simulink model "RoboBoat_NEDcallv8"  (R2014a)
settings: Solver=FixedStepDiscrete  StartTime=0.0  StopTime=inf  FixedStep=.1  RelTol=1e-3
undefined symbols (not defined in the file): Com1, Com2, Com3, Com4, DiscIntNeverNeededParam, standard
libraries: xpcseriallib x31, visiontextngfix x25, simulink x19, slrtlib x9, speedgoatlib_IO102 x3, speedgoatlib x1
(part 2 of 4)

== matlab function RoboBoat_NEDcallv8/Main FSM/Obstacle Navigation1/Obstacle Navigation/MATLAB Function ==
  data: dodgeIncomplete input; dodgeStart input; taskSelector output; dodgeEn output; GPSEn output
function [taskSelector, dodgeEn, GPSEn]  = obstNavEnabler(dodgeIncomplete, dodgeStart)

GPSEn = 0;
dodgeEn = 0;

if  dodgeStart == 1 || dodgeIncomplete == 1
    dodgeEn = 1;
    taskSelector = 1;
else
    GPSEn = 1;
    taskSelector = 2;
end

== matlab function RoboBoat_NEDcallv8/Main FSM/Obstacle Navigation1/GPS: Center/Approach/Desired Heading and Distance ==
  data: Distance output; DesiredGPS input; DesiredHeading output; GPSLat input; GPSLong input
function [Distance, DesiredHeading] = Approach(DesiredGPS, GPSLat, GPSLong)

%Written by Anderson Lebbad on July 22, 2013
%Last Edited: Edward Zhu July 5, 2014

%Edit:
% Switched from great-circle distance formula to equirectangular approx and
%used mod for desired heading
% Changed calculation to use positve lat and negative long

%Orients the boat towards a target GPS point before approaching it.
%This is done to keep the approach angle minimal, so the approach
%algorithm does not circle the target and never reach it.

%Parse input GPS and convert angles to radians
CurLat = (floor(GPSLat/100)+mod(GPSLat,100)/60)*pi/180;
CurLong = (ceil(GPSLong/100)-mod(-GPSLong,100)/60)*pi/180;
DesLat = (floor(DesiredGPS(1)/100)+mod(DesiredGPS(1),100)/60)*pi/180;
DesLong = (ceil(DesiredGPS(2)/100)-mod(-DesiredGPS(2),100)/60)*pi/180;

%Difference between lats and longs
DiffLat = DesLat - CurLat;
MidLat = cos((CurLat + DesLat)/2);
DiffLong = DesLong - CurLong;

%Radius of the earth in meters
R = 6378137;

%Calculate distance using the great-circle distance formula
%Formula documented here:
%   http://www.movable-type.co.uk/scripts/latlong.html
% a = sin(DiffLat/2)^2+sin(DiffLong/2)^2*cos(CurLat)*cos(DesLat);
% c = 2*atan2(sqrt(a), sqrt(1-a));
% Distance = R*c;

%Calculating distance using equirectangular approximation since distances
%concerned are very small
a = DiffLong*MidLat;
b = DiffLat;
Distance = R*sqrt(a^2+b^2);

%Calculate initial bearing - formula documented here: 
%   http://www.movable-type.co.uk/scripts/latlong.html
y = sin(DiffLong)*cos(DesLat);
x = cos(CurLat)*sin(DesLat)-sin(CurLat)*cos(DesLat)*cos(DiffLong);
DesiredHeading = mod(atan2(y, x)*180/pi + 360, 360);

== matlab function RoboBoat_NEDcallv8/Main FSM/Obstacle Navigation1/Obstacle Navigation/GPS: Bee Line/Approach/Desired Heading and Distance ==
  data: Distance output; DesiredGPS input; DesiredHeading output; GPSLat input; GPSLong input
function [Distance, DesiredHeading] = Approach(DesiredGPS, GPSLat, GPSLong)

%Written by Anderson Lebbad on July 22, 2013
%Last Edited: Edward Zhu July 5, 2014

%Edit:
% Switched from great-circle distance formula to equirectangular approx and
%used mod for desired heading
% Changed calculation to use positve lat and negative long

%Orients the boat towards a target GPS point before approaching it.
%This is done to keep the approach angle minimal, so the approach
%algorithm does not circle the target and never reach it.

%Parse input GPS and convert angles to radians
CurLat = (floor(GPSLat/100)+mod(GPSLat,100)/60)*pi/180;
CurLong = (ceil(GPSLong/100)-mod(-GPSLong,100)/60)*pi/180;
DesLat = (floor(DesiredGPS(1)/100)+mod(DesiredGPS(1),100)/60)*pi/180;
DesLong = (ceil(DesiredGPS(2)/100)-mod(-DesiredGPS(2),100)/60)*pi/180;

%Difference between lats and longs
DiffLat = DesLat - CurLat;
MidLat = cos((CurLat + DesLat)/2);
DiffLong = DesLong - CurLong;

%Radius of the earth in meters
R = 6378137;

%Calculate distance using the great-circle distance formula
%Formula documented here:
%   http://www.movable-type.co.uk/scripts/latlong.html
% a = sin(DiffLat/2)^2+sin(DiffLong/2)^2*cos(CurLat)*cos(DesLat);
% c = 2*atan2(sqrt(a), sqrt(1-a));
% Distance = R*c;

%Calculating distance using equirectangular approximation since distances
%concerned are very small
a = DiffLong*MidLat;
b = DiffLat;
Distance = R*sqrt(a^2+b^2);

%Calculate initial bearing - formula documented here: 
%   http://www.movable-type.co.uk/scripts/latlong.html
y = sin(DiffLong)*cos(DesLat);
x = cos(CurLat)*sin(DesLat)-sin(CurLat)*cos(DesLat)*cos(DiffLong);
DesiredHeading = mod(atan2(y, x)*180/pi + 360, 360);

== matlab function RoboBoat_NEDcallv8/Sensors/1020 Comms/Data Update2 ==
  data: Valid input; ControlMode input; V output; C output; L output; A output; Data input; D1 output; D2 output; D3 output; D4 output; D5 output; D6 output; D7 output; D8 output; D9 output; D10 output; D11 output; D12 output; D13 output; D14 output; D15 output; D16 output; D17 output; D18 output; D19 output; D20 output; D21 output; D22 output; D23 output; D24 output; Activate input
function [V,C,L,A,D1,D2,D3,D4,D5,D6,D7,D8,D9,D10,D11,D12,D13,D14,D15,D16,D17,...
    D18,D19,D20,D21,D22,D23,D24] = dataSplit(Valid,ControlMode,Data,Activate)
%Written by Anderson Lebbad on August 10, 2014
%Last Edited by: Anderson Lebbad on September 11, 2014

%This function splits the data vector into the twelve channels it is
%composed of for communication

persistent HoldData

if isempty(HoldData)
    HoldData = zeros(26,1);
    HoldData(2) = 2;
end

if Valid == 1
    HoldData(1) = Valid;
    HoldData(2) = ControlMode;
    HoldData(3) = Data(1);
    HoldData(4) = Data(2);
    HoldData(5) = Data(3);
    HoldData(6) = Data(4);
    HoldData(7) = Data(5);
    HoldData(8) = Data(6);
    HoldData(9) = Data(7);
    HoldData(10) = Data(8);
    HoldData(11) = Data(9);
    HoldData(12) = Data(10);
    HoldData(13) = Data(11);
    HoldData(14) = Data(12);
    HoldData(15) = Data(13);
    HoldData(16) = Data(14);
    HoldData(17) = Data(15);
    HoldData(18) = Data(16);
    HoldData(19) = Data(17);
    HoldData(20) = Data(18);
    HoldData(21) = Data(19);
    HoldData(22) = Data(20);
    HoldData(23) = Data(21);
    HoldData(24) = Data(22);
    HoldData(25) = Data(23);
    HoldData(26) = Data(24);
end

V = HoldData(1);
C = HoldData(2);
L = 8;
A = Activate;
D1 = HoldData(3);
D2 = HoldData(4);
D3 = HoldData(5);
D4 = HoldData(6);
D5 = HoldData(7);
D6 = HoldData(8);
D7 = HoldData(9);
D8 = HoldData(10);
D9 = HoldData(11);
D10 = HoldData(12);
D11 = HoldData(13);
D12 = HoldData(14);
D13 = HoldData(15);
D14 = HoldData(16);
D15 = HoldData(17);
D16 = HoldData(18);
D17 = HoldData(19);
D18 = HoldData(20);
D19 = HoldData(21);
D20 = HoldData(22);
D21 = HoldData(23);
D22 = HoldData(24);
D23 = HoldData(25);
D24 = HoldData(26);

end

== matlab function RoboBoat_NEDcallv8/Sensors/1020 Comms/MATLAB Function3 ==
  data: Time input; asciiHRT output; Lat input; Long input; Mode input; Task input
% This function creates the heartbeat message to be sent from Speedgoat in
% ascii code
% Written by: Edward Zhu
% Date: 9/17/14

function asciiHRT = asciiHRTEncoder(Time, Lat, Long, Mode, Task)

% Initialize output message vector as the serial output block expects 128
% character message
asciiHRT = uint8(zeros(1,128));

% Convert static strings to ascii code
asciiMsgID = uint8('$RXHRT,');
asciiComma = uint8(',');
asciiDeciPt = uint8('.');
if Lat >= 0
    asciiNS = uint8('N,');
else
    Lat = -Lat;
    asciiNS = uint8('S,');
end
if Long >= 0
    asciiEW = uint8('E,');
else
    Long = -Long;
    asciiEW = uint8('W,');
end
asciiTeamID = uint8('FAUVU,');
asciiMsgEnd = uint8('*');
asciiMsgCRLF = [13 10];

% Convert UTC Time input (hhmmss) into ascii code
asciiTime = uint8(zeros(1,7));
asciiTime(7) = asciiComma;

for timeChar = 1:6
    asciiTime(timeChar) = floor(mod(Time,10^(7-timeChar))/...
        10^(6-timeChar)) + 48;
end

% Convert latitude (dd.mmmmmm) into ascii code
asciiLat = uint8(zeros(1,10));
asciiLat(10) = asciiComma;
asciiLat(3) = asciiDeciPt;

latInt = floor(Lat);
for latIntChar = 1:2
    asciiLat(latIntChar) = floor(mod(latInt,10^(3-latIntChar))/...
        10^(2-latIntChar)) + 48;
end

latDeci = mod(Lat,latInt) * 10^6;
for latDeciChar = 1:6
    asciiLat(latDeciChar+3) = floor(mod(latDeci,10^(7-latDeciChar))/...
        10^(6-latDeciChar)) + 48;
end

% Convert longitude (ddd.mmmmmm) into ascii code
asciiLong = uint8(zeros(1,11));
asciiLong(11) = asciiComma;
asciiLong(4) = asciiDeciPt;

longInt = floor(Long);
for longIntChar = 1:3
    asciiLong(longIntChar) = floor(mod(longInt,10^(4-longIntChar))/...
        10^(3-longIntChar)) + 48;
end

longDeci = mod(Long,longInt) * 10^6;
for longDeciChar = 1:6
    asciiLong(longDeciChar+4) = floor(mod(longDeci,10^(7-longDeciChar))/...
        10^(6-longDeciChar)) + 48;
end

% Convert vehicle mode into ascii (1 = RC, 2 = Auto)
if Mode ~= 1 || Mode ~= 2
    Mode = 1;
    asciiMode = [uint8(Mode+48) asciiComma];
else
    asciiMode = [uint8(Mode+48) asciiComma];
end

% Convert vehicle task into ascii
asciiTask = [uint8(Task+48) asciiMsgEnd];

% Concat individual ascii arrays into one array
asciiPreChkSum = cat(2,asciiMsgID,asciiTime,asciiLat,asciiNS,asciiLong,asciiEW,...
    asciiTeamID,asciiMode,asciiTask);

% Calculate the checksum of the message from the '$' to the '*' and convert
% to hex
chkSum = uint8(0);

for chksumChar = 1:(length(asciiPreChkSum)-2)
    chkSum = bitxor(chkSum,asciiPreChkSum(chksumChar+1));
end

% Convert the checksum to ascii
chkSum = dec2hex(chkSum);
asciiChkSum = uint8(zeros(1,length(chkSum))+32);
for i = 1:length(chkSum)
    asciiChkSum(i) = uint8(chkSum(i));
end

% Concat the checksum and the '/r/n' to the end of the message
asciiPostChkSum = cat(2,asciiPreChkSum,asciiChkSum,asciiMsgCRLF);

% Output the final message
asciiHRT(1:length(asciiPostChkSum)) = asciiPostChkSum;

== system RoboBoat_NEDcallv8/Sensors/1020 Comms/ Raspberry Pi LCM (Navigation and Acoustics) ==
  LCM Input : Inport
  ASCII Decode 6 : xpcseriallib/ASCII Decode   format=P1:%f P2:%f P3:%f V1:%f V2:%f V3:%f E1:%f E2:%f E3:%f Pt1:%f Pt2:%f St1:%f St2:%f Start:%f Elapsed:%f RC:%d Deploy:%u, Elapsed:%g, Bearing1:%g Bearing2:%g \r\n  nvars=22  vartypes={}
  Bus Creator{,5..7} (4 alike) : BusCreator  Inputs=2
  Bus Creator{1..3,8} (4 alike) : BusCreator  Inputs=3
  Bus Creator4 : BusCreator  Inputs=9
  Data Type Conversion : DataTypeConversion  OutDataTypeStr=double
  FIFO ASCII read 1 : xpcseriallib/FIFO ASCII read   header={'P1:'}  term=[13 10]  hold=Zero output if no new data  enable=off  maxsize=2048  outputtype=8 bit uint null terminated  sampletime=-1
  Navigation LCM : Outport
  Acoustic LCM : Outport  Port=2
  wires:
  LCM Input/1 -> FIFO ASCII read 1/1
  FIFO ASCII read 1/1 -> ASCII Decode 6/1
  Bus Creator4/1 -> Navigation LCM/1  "Navigation Message"
  ASCII Decode 6/1 -> Bus Creator1/1  "X"
  ASCII Decode 6/2 -> Bus Creator1/2  "Y"
  ASCII Decode 6/3 -> Bus Creator1/3  "Psi"
  Bus Creator1/1 -> Bus Creator4/1  "Pose"
  ASCII Decode 6/4 -> Bus Creator2/1  "u"
  ASCII Decode 6/5 -> Bus Creator2/2  "v"
  Bus Creator2/1 -> Bus Creator4/2  "Velocity"
  ASCII Decode 6/7 -> Bus Creator3/1  "Roll"
  ASCII Decode 6/8 -> Bus Creator3/2  "Pitch"
  ASCII Decode 6/9 -> Bus Creator3/3  "Yaw"
  Bus Creator3/1 -> Bus Creator4/3  "Euler"
  Bus Creator5/1 -> Bus Creator4/5  "Port"
  Bus Creator6/1 -> Bus Creator4/6  "Stbd"
  ASCII Decode 6/14 -> Bus Creator6/1  "StThrust"
  ASCII Decode 6/15 -> Bus Creator6/2  "StAzimuth"
  ASCII Decode 6/12 -> Bus Creator5/1  "PtThrust"
  ASCII Decode 6/13 -> Bus Creator5/2  "PtAzimuth"
  ASCII Decode 6/16 -> Bus Creator4/7  "Start"
  ASCII Decode 6/17 -> Bus Creator4/8  "Elapsed"
  ASCII Decode 6/18 -> Data Type Conversion/1  "On/Off/RC/Auto"
  Data Type Conversion/1 -> Bus Creator4/9  "On/Off/RC/Auto"
  ASCII Decode 6/6 -> Bus Creator2/3  "r"
  ASCII Decode 6/10 -> Bus Creator7/1  "Lat"
  ASCII Decode 6/11 -> Bus Creator7/2  "Long"
  Bus Creator7/1 -> Bus Creator4/4  "GPS (LLA)"
  ASCII Decode 6/21 -> Bus Creator/1  "Horizontal Bearing"
  ASCII Decode 6/22 -> Bus Creator/2  "Vertical Bearing"
  Bus Creator/1 -> Bus Creator8/3  "Bearings"
  ASCII Decode 6/20 -> Bus Creator8/2  "Elapsed Time"
  ASCII Decode 6/19 -> Bus Creator8/1  "Deployed"
  Bus Creator8/1 -> Acoustic LCM/1  "Acoustic Message"

== system RoboBoat_NEDcallv8/Sensors/1020 Comms/ Raspberry Pi LCM (Navigation) ==
  LCM Input : Inport
  ASCII Decode 6 : xpcseriallib/ASCII Decode   format=P1:%f P2:%f P3:%f V1:%f V2:%f V3:%f E1:%f E2:%f E3:%f Lat:%f Long:%f Pt1:%f Pt2:%f St1:%f St2:%f Start:%f Elapsed:%f RC:%d Deploy:%u Elapsed:%f Bearing1:%f Bearing2:%f Range:%f X_Pos:%f Y_Pos:%f \r\n  nvars=25  vartypes={}
  Bus Creator1 : BusCreator  Inputs=3
  Bus Creator2 : BusCreator  Inputs=3
  Bus Creator3 : BusCreator  Inputs=3
  Bus Creator4 : BusCreator  Inputs=9
  Bus Creator5 : BusCreator  Inputs=2
  Bus Creator6 : BusCreator  Inputs=2
  Bus Creator7 : BusCreator  Inputs=2
  Bus Creator8 : BusCreator  Inputs=7
  Data Type Conversion : DataTypeConversion  OutDataTypeStr=double
  FIFO ASCII read 1 : xpcseriallib/FIFO ASCII read   header={'P1:'}  term=[13 10]  hold=Zero output if no new data  enable=off  maxsize=2000  outputtype=8 bit uint null terminated  sampletime=-1
  LCM Output : Outport
  Acou LCM : Outport  Port=2
  wires:
  LCM Input/1 -> FIFO ASCII read 1/1
  FIFO ASCII read 1/1 -> ASCII Decode 6/1
  Bus Creator4/1 -> LCM Output/1  "Navigation Message"
  ASCII Decode 6/1 -> Bus Creator1/1  "X"
  ASCII Decode 6/2 -> Bus Creator1/2  "Y"
  ASCII Decode 6/3 -> Bus Creator1/3  "Psi"
  Bus Creator1/1 -> Bus Creator4/1  "Pose"
  ASCII Decode 6/4 -> Bus Creator2/1  "u"
  ASCII Decode 6/5 -> Bus Creator2/2  "v"
  Bus Creator2/1 -> Bus Creator4/2  "Velocity"
  ASCII Decode 6/7 -> Bus Creator3/1  "Roll"
  ASCII Decode 6/8 -> Bus Creator3/2  "Pitch"
  ASCII Decode 6/9 -> Bus Creator3/3  "Yaw"
  Bus Creator3/1 -> Bus Creator4/3  "Euler"
  Bus Creator5/1 -> Bus Creator4/5  "Port"
  Bus Creator6/1 -> Bus Creator4/6  "Stbd"
  ASCII Decode 6/14 -> Bus Creator6/1  "StThrust"
  ASCII Decode 6/15 -> Bus Creator6/2  "StAzimuth"
  ASCII Decode 6/12 -> Bus Creator5/1  "PtThrust"
  ASCII Decode 6/13 -> Bus Creator5/2  "PtAzimuth"
  ASCII Decode 6/16 -> Bus Creator4/7  "Start"
  ASCII Decode 6/17 -> Bus Creator4/8  "Elapsed"
  ASCII Decode 6/18 -> Data Type Conversion/1  "On/Off/RC/Auto"
  Data Type Conversion/1 -> Bus Creator4/9  "On/Off/RC/Auto"
  ASCII Decode 6/6 -> Bus Creator2/3  "r"
  ASCII Decode 6/10 -> Bus Creator7/1  "Lat"
  ASCII Decode 6/11 -> Bus Creator7/2  "Long"
  Bus Creator7/1 -> Bus Creator4/4  "GPS (LLA)"
  ASCII Decode 6/19 -> Bus Creator8/1  "Deployed"
  ASCII Decode 6/20 -> Bus Creator8/2  "Elapsed Time"
  ASCII Decode 6/21 -> Bus Creator8/3  "Horizontal Bearing"
  ASCII Decode 6/22 -> Bus Creator8/4  "Vertical Bearing"
  ASCII Decode 6/23 -> Bus Creator8/5  "Range"
  ASCII Decode 6/24 -> Bus Creator8/6  "X Pos"
  ASCII Decode 6/25 -> Bus Creator8/7  "Y Pos"
  Bus Creator8/1 -> Acou LCM/1

== system RoboBoat_NEDcallv8/Sensors/1020 Comms/Acoustic LCM ==
  LCM Input : Inport
  Bus Creator : BusCreator  Inputs=2
  Bus Creator1 : BusCreator
  Bus Creator2 : BusCreator  Inputs=3
  Bus Selector : BusSelector  OutputSignals=Deployed,Elapsed Time,Horizontal Bearing,Vertical Bearing,Range,X Pos,Y Pos
  LCM Output : Outport
  wires:
  Bus Selector/3 -> Bus Creator/1  "<Horizontal Bearing>"
  Bus Selector/4 -> Bus Creator/2  "<Vertical Bearing>"
  Bus Creator/1 -> Bus Creator1/3  "Bearings"
  Bus Selector/2 -> Bus Creator1/2  "<Elapsed Time>"
  Bus Selector/1 -> Bus Creator1/1  "<Deployed>"
  Bus Creator1/1 -> LCM Output/1  "Acoustic Message"
  LCM Input/1 -> Bus Selector/1
  Bus Selector/5 -> Bus Creator2/1  "<Range>"
  Bus Selector/6 -> Bus Creator2/2  "<X Pos>"
  Bus Selector/7 -> Bus Creator2/3  "<Y Pos>"
  Bus Creator2/1 -> Bus Creator1/4  "Pose Estimate"

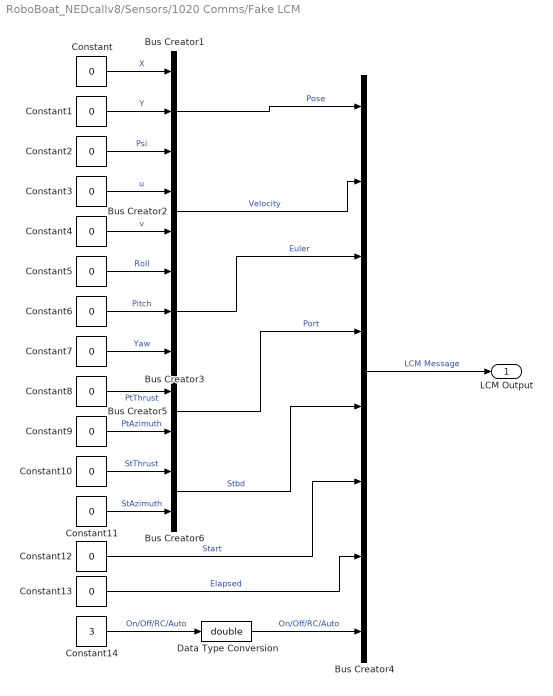
== system RoboBoat_NEDcallv8/Sensors/1020 Comms/Fake LCM ==
  Bus Creator1 : BusCreator  Inputs=3
  Bus Creator2 : BusCreator  Inputs=2
  Bus Creator3 : BusCreator  Inputs=3
  Bus Creator4 : BusCreator  Inputs=8
  Bus Creator5 : BusCreator  Inputs=2
  Bus Creator6 : BusCreator  Inputs=2
  Constant{,1..13} (14 alike) : Constant  Value=0
  Constant14 : Constant  Value=3
  Data Type Conversion : DataTypeConversion  OutDataTypeStr=double
  LCM Output : Outport
  wires:
  Bus Creator4/1 -> LCM Output/1  "LCM Message"
  Constant/1 -> Bus Creator1/1  "X"
  Constant1/1 -> Bus Creator1/2  "Y"
  Constant2/1 -> Bus Creator1/3  "Psi"
  Bus Creator1/1 -> Bus Creator4/1  "Pose"
  Constant3/1 -> Bus Creator2/1  "u"
  Constant4/1 -> Bus Creator2/2  "v"
  Bus Creator2/1 -> Bus Creator4/2  "Velocity"
  Constant5/1 -> Bus Creator3/1  "Roll"
  Constant6/1 -> Bus Creator3/2  "Pitch"
  Constant7/1 -> Bus Creator3/3  "Yaw"
  Bus Creator3/1 -> Bus Creator4/3  "Euler"
  Bus Creator5/1 -> Bus Creator4/4  "Port"
  Bus Creator6/1 -> Bus Creator4/5  "Stbd"
  Constant10/1 -> Bus Creator6/1  "StThrust"
  Constant11/1 -> Bus Creator6/2  "StAzimuth"
  Constant8/1 -> Bus Creator5/1  "PtThrust"
  Constant9/1 -> Bus Creator5/2  "PtAzimuth"
  Constant12/1 -> Bus Creator4/6  "Start"
  Constant13/1 -> Bus Creator4/7  "Elapsed"
  Constant14/1 -> Data Type Conversion/1  "On/Off/RC/Auto"
  Data Type Conversion/1 -> Bus Creator4/8  "On/Off/RC/Auto"

== system RoboBoat_NEDcallv8/Sensors/1020 Comms/LIDAR Panda ==
  LIDAR Panda In : Inport
  ASCII Decode 2 : xpcseriallib/ASCII Decode   format=A:%d B:%d C:%d E:%d F:%d G:%d H:%d I:%d J:%d K:%d L:%d M:%d N:%d O:%d P:%d Q:%d R:%d S:%d T:%d U:%d V:%d W:%d X:%d C1:%d C2:%d C3:%d C4:%d P1:%f P2:%f P3:%f P4:%f I1:%d I2:%d I3:%d I4:%d \r\n  nvars=36  vartypes={}
  Bus Creator1 : BusCreator  Inputs=2
  Bus Creator2 : BusCreator  Inputs=3
  Bus Creator3 : BusCreator  Inputs=2
  Data Type Conversion{,1..3} (4 alike) : DataTypeConversion  OutDataTypeStr=double
  "FIFO ASCII read " : xpcseriallib/FIFO ASCII read   header={'A:'}  term=[13 10]  hold=Zero output if no new data  enable=off  maxsize=1024  outputtype=8 bit uint null terminated  sampletime=-1
  Mux : Mux  Inputs=12
  Mux1 : Mux
  Mux2 : Mux  Inputs=12
  Mux3 : Mux
  Mux4 : Mux
  LIDAR Panda Out : Outport
  wires:
  LIDAR Panda In/1 -> "FIFO ASCII read "/1
  "FIFO ASCII read "/1 -> ASCII Decode 2/1
  ASCII Decode 2/3 -> Mux/3  "Distance"
  ASCII Decode 2/2 -> Mux/2  "Color ID"
  ASCII Decode 2/4 -> Mux/4  "Angle"
  ASCII Decode 2/1 -> Mux/1  "Probability"
  ASCII Decode 2/7 -> Mux/7
  ASCII Decode 2/10 -> Mux/10
  ASCII Decode 2/11 -> Mux/11
  ASCII Decode 2/6 -> Mux/6
  ASCII Decode 2/8 -> Mux/8
  ASCII Decode 2/9 -> Mux/9
  ASCII Decode 2/12 -> Mux/12
  ASCII Decode 2/5 -> Mux/5
  ASCII Decode 2/13 -> Mux2/1
  ASCII Decode 2/15 -> Mux2/3
  ASCII Decode 2/22 -> Mux2/10
  ASCII Decode 2/23 -> Mux2/11
  ASCII Decode 2/17 -> Mux2/5
  ASCII Decode 2/18 -> Mux2/6
  ASCII Decode 2/14 -> Mux2/2
  ASCII Decode 2/24 -> Mux2/12
  ASCII Decode 2/20 -> Mux2/8
  ASCII Decode 2/19 -> Mux2/7
  ASCII Decode 2/21 -> Mux2/9
  ASCII Decode 2/16 -> Mux2/4
  ASCII Decode 2/25 -> Mux1/1
  ASCII Decode 2/28 -> Mux1/4
  ASCII Decode 2/26 -> Mux1/2
  ASCII Decode 2/27 -> Mux1/3
  ASCII Decode 2/30 -> Mux3/2
  ASCII Decode 2/31 -> Mux3/3
  ASCII Decode 2/32 -> Mux3/4
  ASCII Decode 2/29 -> Mux3/1
  ASCII Decode 2/36 -> Mux4/4
  ASCII Decode 2/34 -> Mux4/2
  ASCII Decode 2/35 -> Mux4/3
  ASCII Decode 2/33 -> Mux4/1
  Mux/1 -> Data Type Conversion/1  "Distances"
  Mux2/1 -> Data Type Conversion1/1  "Angles"
  Mux1/1 -> Data Type Conversion2/1  "Color"
  Mux3/1 -> Bus Creator2/2  "Probability"
  Mux4/1 -> Data Type Conversion3/1  "idx"
  Bus Creator1/1 -> Bus Creator3/1  "Landmarks"
  Bus Creator2/1 -> Bus Creator3/2  "Color data"
  Bus Creator3/1 -> LIDAR Panda Out/1
  Data Type Conversion/1 -> Bus Creator1/1  "Distances"
  Data Type Conversion1/1 -> Bus Creator1/2  "Angles"
  Data Type Conversion2/1 -> Bus Creator2/1  "Color"
  Data Type Conversion3/1 -> Bus Creator2/3  "Color"

== system RoboBoat_NEDcallv8/Sensors/1020 Comms/Subsystem ==
  Bus Creator : BusCreator  Inputs=3
  Bus Creator1 : BusCreator  Inputs=2
  Bus Creator2 : BusCreator  Inputs=2
  Constant : Constant  Value=zeros(12,1)
  Constant1 : Constant  Value=zeros(12,1)
  Constant2 : Constant  Value=zeros(4,1)
  Constant3 : Constant  Value=zeros(4,1)
  Constant4 : Constant  Value=zeros(4,1)
  Fake Panda : Outport
  wires:
  Constant/1 -> Bus Creator1/1  "Distances"
  Constant1/1 -> Bus Creator1/2  "Angles"
  Constant2/1 -> Bus Creator/1  "Color"
  Constant3/1 -> Bus Creator/2  "Probability"
  Constant4/1 -> Bus Creator/3  "idx"
  Bus Creator1/1 -> Bus Creator2/1  "Landmarks"
  Bus Creator/1 -> Bus Creator2/2  "Color data"
  Bus Creator2/1 -> Fake Panda/1  "Lidar Data Input"

== system RoboBoat_NEDcallv8/Sensors/1020 Comms/data log ==
  Sensors signal : Inport
  Bus Selector3 : BusSelector  OutputSignals=Navigation Message,Lidar Data Input,Acoustic Message
  Bus to Vector : BusToVector
  Bus to Vector1 : BusToVector
  Bus to Vector2 : BusToVector
  Read : DataStoreRead  DataStoreName=PingPose
  Scope 1 : slrtlib/Displays and Logging/Scope   scopeno=3  scopetype=File  autostart=on  viewmode=Graphical redraw  formatstr='%15.6f'  grid=on  ylimits=[0,0]  nosamples=28800  noprepostsamples=0  interleave=1  triggermode=FreeRun  triggersignal=1  trigsignalfromport=off  triggerlevel=0.0  triggerslope=Either  triggerscope=1  triggersample=0  filename=LM1_<%%%>.dat  mode=Lazy  writesize=5120  autorestart=on  dynamicfilemode=on  maxwritefilesize=512*1024^2
  Scope 2 : slrtlib/Displays and Logging/Scope   scopeno=1  scopetype=File  autostart=on  viewmode=Graphical redraw  formatstr='%15.6f'  grid=on  ylimits=[0,0]  nosamples=28800  noprepostsamples=0  interleave=1  triggermode=FreeRun  triggersignal=1  trigsignalfromport=off  triggerlevel=0.0  triggerslope=Either  triggerscope=1  triggersample=0  filename=NAV1_<%%%>.dat  mode=Lazy  writesize=5120  autorestart=on  dynamicfilemode=on  maxwritefilesize=512*1024^2
  Scope 3 : slrtlib/Displays and Logging/Scope   scopeno=2  scopetype=File  autostart=on  viewmode=Graphical redraw  formatstr='%15.6f'  grid=on  ylimits=[0,0]  nosamples=28800  noprepostsamples=0  interleave=1  triggermode=FreeRun  triggersignal=1  trigsignalfromport=off  triggerlevel=0.0  triggerslope=Either  triggerscope=1  triggersample=0  filename=ACO1_<%%%>.dat  mode=Lazy  writesize=5120  autorestart=on  dynamicfilemode=on  maxwritefilesize=512*1024^2
  Scope 4 : slrtlib/Displays and Logging/Scope   scopeno=4  scopetype=File  autostart=on  viewmode=Graphical redraw  formatstr='%15.6f'  grid=on  ylimits=[0,0]  nosamples=28800  noprepostsamples=0  interleave=1  triggermode=FreeRun  triggersignal=1  trigsignalfromport=off  triggerlevel=0.0  triggerslope=Either  triggerscope=1  triggersample=0  filename=pPos_<%%%>.dat  mode=Lazy  writesize=5120  autorestart=on  dynamicfilemode=on  maxwritefilesize=512*1024^2
  wires:
  Sensors signal/1 -> Bus Selector3/1
  Bus to Vector/1 -> Scope 2/1
  Bus Selector3/1 -> Bus to Vector/1  "<Navigation Message>"
  Bus to Vector1/1 -> Scope 1/1
  Bus to Vector2/1 -> Scope 3/1
  Bus Selector3/3 -> Bus to Vector2/1  "<Acoustic Message>"
  Bus Selector3/2 -> Bus to Vector1/1  "<Lidar Data Input>"
  Read/1 -> Scope 4/1

== system RoboBoat_NEDcallv8/Sensors/Baseboard Serial/Compass Decode ==
  note: Status Field can be one of the following:
      | L = low alarm
      | M= low warning
      | N = Normal
      | O = High Warning
      | P = High Alarm
      | C = Tuning analog circuit
  note: Compas NMEA- Raw data from the Compass
  Compass NMEA : Inport
  "ASCII Decode " : xpcseriallib/ASCII Decode   format=$PTNTHPR,%f,%c%f,%c%f,%c  nvars=7  vartypes={ }
  Bus Creator : BusCreator  Inputs=3
  Correct Heading Angle Magnetic to True North : Subsystem
  "FIFO ASCII read " : xpcseriallib/FIFO ASCII read   header={'$PTNTHPR'}  term=[13 10]  hold=Zero output if no new data  enable=off  maxsize=64  outputtype=8 bit uint null terminated  sampletime=-1
  Terminator{,1..3} (4 alike) : Terminator
  Compass data (3) : Outport
  wires:
  "FIFO ASCII read "/1 -> "ASCII Decode "/1
  Compass NMEA/1 -> "FIFO ASCII read "/1
  "ASCII Decode "/2 -> Terminator/1
  "ASCII Decode "/4 -> Terminator1/1
  "ASCII Decode "/6 -> Terminator2/1
  "ASCII Decode "/7 -> Terminator3/1
  Bus Creator/1 -> Compass data (3)/1  "Compass"
  "ASCII Decode "/3 -> Bus Creator/2  "Pitch"
  "ASCII Decode "/5 -> Bus Creator/3  "Roll"
  "ASCII Decode "/1 -> Correct Heading Angle Magnetic to True North/1(Heading Mag)  "Heading"
  Correct Heading Angle Magnetic to True North/1(Heading True) -> Bus Creator/1  "Heading"

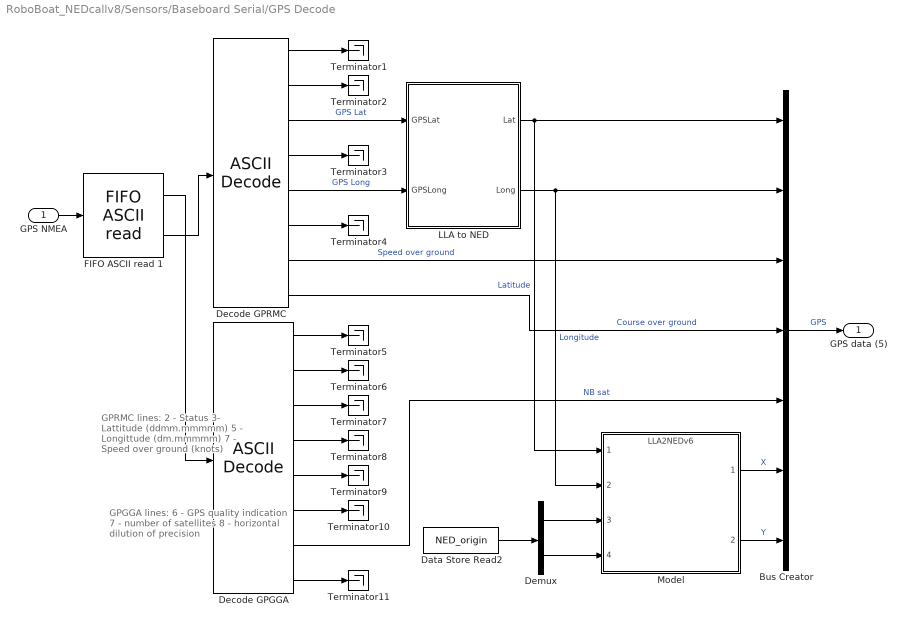
== system RoboBoat_NEDcallv8/Sensors/Baseboard Serial/GPS Decode ==
  note: GPGGA lines:
      | 6 - GPS quality indication
      | 7 - number of satellites
      | 8 - horizontal dilution of precision
  note: GPRMC lines:
      | 2 - Status
      | 3- Lattitude (ddmm.mmmmm)
      | 5 - Longittude (dm.mmmmm)
      | 7 - Speed over ground (knots)
  GPS NMEA : Inport
  Bus Creator : BusCreator  Inputs=7
  Data Store Read2 : DataStoreRead  DataStoreName=NED_origin
  Decode GPGGA : xpcseriallib/ASCII Decode   format=$GPGGA,%d,%f,%c%f,%c%f,%f,%f  nvars=8  vartypes={ }
  Decode GPRMC : xpcseriallib/ASCII Decode   format=$GPRMC,%f,%c%f,%c%f,%c%f,%f  nvars=8  vartypes={ }
  Demux : Demux  Outputs=2
  FIFO ASCII read 1 : xpcseriallib/FIFO ASCII read   header={'$GPGGA','$GPRMC'}  term=[13 10]  hold=Zero output if no new data  enable=off  maxsize=1024  outputtype=8 bit uint null terminated  sampletime=-1
  LLA to NED : MATLAB Function  TreatAsAtomicUnit=on
  Model : ModelReference  ModelNameDialog=LLA2NEDv6.slx  SimulationMode=Normal  ModelReferenceVersion=1.2057  CopyOfModelName=LLA2NEDv6.slx  DefaultDataLogging=on
  Terminator{1..11} (11 alike) : Terminator
  GPS data (5) : Outport
  wires:
  Decode GPRMC/1 -> Terminator1/1
  Decode GPRMC/7 -> Bus Creator/3  "Speed over ground"
  GPS NMEA/1 -> FIFO ASCII read 1/1
  FIFO ASCII read 1/1 -> Decode GPGGA/1
  FIFO ASCII read 1/2 -> Decode GPRMC/1
  Decode GPRMC/8 -> Bus Creator/4  "Course over ground"
  Decode GPGGA/7 -> Bus Creator/5  "NB sat"
  Decode GPRMC/2 -> Terminator2/1
  Decode GPRMC/4 -> Terminator3/1
  Decode GPRMC/6 -> Terminator4/1
  Decode GPGGA/1 -> Terminator5/1
  Decode GPGGA/2 -> Terminator6/1
  Decode GPGGA/3 -> Terminator7/1
  Decode GPGGA/4 -> Terminator8/1
  Decode GPGGA/5 -> Terminator9/1
  Decode GPGGA/6 -> Terminator10/1
  Decode GPGGA/8 -> Terminator11/1
  Bus Creator/1 -> GPS data (5)/1  "GPS"
  Model/1 -> Bus Creator/6  "X"
  Model/2 -> Bus Creator/7  "Y"
  Decode GPRMC/3 -> LLA to NED/1(GPSLat)  "GPS Lat"
  Decode GPRMC/5 -> LLA to NED/2(GPSLong)  "GPS Long"
  LLA to NED/1(Lat) -> Model/1, Bus Creator/1  "Latitude"
  LLA to NED/2(Long) -> Model/2, Bus Creator/2  "Longitude"
  Data Store Read2/1 -> Demux/1
  Demux/1 -> Model/3
  Demux/2 -> Model/4

== system RoboBoat_NEDcallv8/Sensors/Baseboard Serial/LIDAR Panda ==
  LIDAR Panda In : Inport
  ASCII Decode 2 : xpcseriallib/ASCII Decode   format=A:%d B:%d C:%d D:%d E:%d F:%d G:%d H:%d I:%d J:%d K:%d L:%d M:%d N:%d O:%d P:%d Q:%d R:%d S:%d T:%d U:%d V:%d W:%d X:%d C1:%d C2:%d C3:%d C4:%d P1:%f P2:%f P3:%f P4:%f I1:%d I2:%d I3:%d I4:%d \r\n  nvars=36  vartypes={}
  Bus Creator1 : BusCreator  Inputs=2
  Bus Creator2 : BusCreator  Inputs=3
  Bus Creator3 : BusCreator  Inputs=2
  Data Type Conversion{,1..3} (4 alike) : DataTypeConversion  OutDataTypeStr=double
  "FIFO ASCII read " : xpcseriallib/FIFO ASCII read   header={'A:'}  term=[13 10]  hold=Zero output if no new data  enable=off  maxsize=1024  outputtype=8 bit uint null terminated  sampletime=-1
  Mux : Mux  Inputs=12
  Mux1 : Mux
  Mux2 : Mux  Inputs=12
  Mux3 : Mux
  Mux4 : Mux
  LIDAR Panda Out : Outport
  wires:
  LIDAR Panda In/1 -> "FIFO ASCII read "/1
  "FIFO ASCII read "/1 -> ASCII Decode 2/1
  ASCII Decode 2/3 -> Mux/3  "Distance"
  ASCII Decode 2/2 -> Mux/2  "Color ID"
  ASCII Decode 2/4 -> Mux/4  "Angle"
  ASCII Decode 2/1 -> Mux/1  "Probability"
  ASCII Decode 2/7 -> Mux/7
  ASCII Decode 2/10 -> Mux/10
  ASCII Decode 2/11 -> Mux/11
  ASCII Decode 2/6 -> Mux/6
  ASCII Decode 2/8 -> Mux/8
  ASCII Decode 2/9 -> Mux/9
  ASCII Decode 2/12 -> Mux/12
  ASCII Decode 2/5 -> Mux/5
  ASCII Decode 2/13 -> Mux2/1
  ASCII Decode 2/15 -> Mux2/3
  ASCII Decode 2/22 -> Mux2/10
  ASCII Decode 2/23 -> Mux2/11
  ASCII Decode 2/17 -> Mux2/5
  ASCII Decode 2/18 -> Mux2/6
  ASCII Decode 2/14 -> Mux2/2
  ASCII Decode 2/24 -> Mux2/12
  ASCII Decode 2/20 -> Mux2/8
  ASCII Decode 2/19 -> Mux2/7
  ASCII Decode 2/21 -> Mux2/9
  ASCII Decode 2/16 -> Mux2/4
  ASCII Decode 2/25 -> Mux1/1
  ASCII Decode 2/28 -> Mux1/4
  ASCII Decode 2/26 -> Mux1/2
  ASCII Decode 2/27 -> Mux1/3
  ASCII Decode 2/30 -> Mux3/2
  ASCII Decode 2/31 -> Mux3/3
  ASCII Decode 2/32 -> Mux3/4
  ASCII Decode 2/29 -> Mux3/1
  ASCII Decode 2/36 -> Mux4/4
  ASCII Decode 2/34 -> Mux4/2
  ASCII Decode 2/35 -> Mux4/3
  ASCII Decode 2/33 -> Mux4/1
  Mux/1 -> Data Type Conversion/1  "Distances"
  Mux2/1 -> Data Type Conversion1/1  "Angles"
  Mux1/1 -> Data Type Conversion2/1  "Color"
  Mux3/1 -> Bus Creator2/2  "Probability"
  Mux4/1 -> Data Type Conversion3/1  "idx"
  Bus Creator1/1 -> Bus Creator3/1  "Landmarks"
  Bus Creator2/1 -> Bus Creator3/2  "Color data"
  Bus Creator3/1 -> LIDAR Panda Out/1
  Data Type Conversion/1 -> Bus Creator1/1  "Distances"
  Data Type Conversion1/1 -> Bus Creator1/2  "Angles"
  Data Type Conversion2/1 -> Bus Creator2/1  "Color"
  Data Type Conversion3/1 -> Bus Creator2/3  "idx"

== system RoboBoat_NEDcallv8/Sinks/actuators/analog output ==
  Compass Heading : Inport
  Control Signals : Inport  Port=2
  Analog output : speedgoatlib_IO102/Analog output  id=1  channels=[1,2,3,4]  range=2  ts=-1  pciSlot=-1
  Ground : Ground
  Subsystem : Subsystem
  wires:
  Subsystem/1(Propulsion) -> Analog output/1
  Subsystem/2(Steering) -> Analog output/2
  Control Signals/1 -> Subsystem/2(Control Signals)
  Compass Heading/1 -> Subsystem/1(Compass Heading)
  Ground/1 -> Analog output/4, Analog output/3

== system RoboBoat_NEDcallv8/Main FSM/Obstacle Navigation1/Communication/Output Heirarchy1 ==
  Desired Heading : Inport
  Sensors : Inport  Port=2
  Annotated Image : Inport  Port=3
  Bus Creator : BusCreator  Inputs=3
  Bus Creator1 : BusCreator  Inputs=2
  Bus Creator2 : BusCreator  Inputs=3
  Bus Creator3 : BusCreator  Inputs=2
  Bus Creator4 : BusCreator  Inputs=2
  Due Sample Start : Constant  Value=0
  Finished : Constant  Value=0
  RPM Desired : Constant  Value=0
  Ready to Read : Constant  Value=0
  Uno Power : Constant  Value=0
  Outputs : Outport
  wires:
  RPM Desired/1 -> Bus Creator/1  "RPM"
  Bus Creator/1 -> Bus Creator1/1  "Control Signals"
  Bus Creator2/1 -> Bus Creator/3  "Arduino Signals"
  Uno Power/1 -> Bus Creator2/2  "Uno Power"
  Desired Heading/1 -> Bus Creator/2  "Desired Heading"
  Bus Creator1/1 -> Bus Creator4/1  "Outputs"
  Annotated Image/1 -> Bus Creator1/2  "Annotated Image"
  Sensors/1 -> Bus Creator4/2  "Sensors"
  Bus Creator4/1 -> Bus Creator3/1  "Output Signals"
  Ready to Read/1 -> Bus Creator2/1  "Ready to Read"
  Due Sample Start/1 -> Bus Creator2/3  "Due Sample Start"
  Bus Creator3/1 -> Outputs/1
  Finished/1 -> Bus Creator3/2  "Task Finished"

== system RoboBoat_NEDcallv8/Main FSM/Obstacle Navigation1/Enter Gate/Gate 1 (Red & White) ==
  Sensors : Inport
  RGB image : Inport  Port=2
  Enable : EnablePort  ShowOutputPort=on
  Bus Selector : BusSelector  OutputSignals=Serial In.Buoy Info.Probability,Serial In.Buoy Info.Color ID,Serial In.Buoy Info.Distance,Serial In.Buoy Info.Angle,Serial In.Compass.Heading,Serial In.GPS.latitude,Serial In.GPS.longitude
  Compare To Constant : simulink/Logic and Bit Operations/Compare To Constant  relop=<=  const=2  OutDataTypeStr=boolean
  Compare To Constant1 : simulink/Logic and Bit Operations/Compare To Constant  relop=>=  const=120  OutDataTypeStr=boolean
  Data Type Conversion2 : DataTypeConversion  OutDataTypeStr=double
  Discrete-Time Integrator : DiscreteIntegrator  SampleTime=.1  ICPrevOutput=DiscIntNeverNeededParam  ICPrevScaledInput=DiscIntNeverNeededParam
  Distance : MATLAB Function  TreatAsAtomicUnit=on
  Insert Text : visiontextngfix/Insert Text  inputType=Obsolete  theText='Enter Gate 1'  getTextLocFrom=Specify via dialog  textLoc=[1 1]  getTextColorFrom=Specify via dialog  textColor=[0 0 0]  getTextIntensityFrom=Specify via dialog  textIntensity=0  getTextOpacityFrom=Specify via dialog  textOpacity=1.0  dummyVar2=0  dummyVar3=0  dummyVar4=0  imagePorts=One multidimensional signal  isInputTransposed=off  fontFace=LucidaSansRegular  dummyVar1=0  blockFontSize=12  antiAliased=on
  Logical Operator : Logic  Operator=OR  AllPortsSameDT=off  OutDataTypeStr=boolean
  MATLAB Function : MATLAB Function  TreatAsAtomicUnit=on
  Output Heirarchy : Subsystem
  Outputs : Outport
  wires:
  Output Heirarchy/1(Outputs) -> Outputs/1
  Sensors/1 -> Output Heirarchy/2(Sensors), Bus Selector/1
  Bus Selector/1 -> MATLAB Function/1(Prob)  "<Probability>"
  Bus Selector/2 -> MATLAB Function/2(ColorID)  "<Color ID>"
  Bus Selector/3 -> MATLAB Function/3(Dist)  "<Distance>"
  Bus Selector/4 -> MATLAB Function/4(Ang)  "<Angle>"
  Bus Selector/5 -> MATLAB Function/5(CurrentHeading)  "<Heading>"
  Enable/1 -> Discrete-Time Integrator/1
  Discrete-Time Integrator/1 -> Compare To Constant1/1, MATLAB Function/8(Timer)
  MATLAB Function/1(RPM) -> Output Heirarchy/3(RPM)
  MATLAB Function/2(DesiredHeading) -> Output Heirarchy/4(Desired Heading)
  Bus Selector/6 -> MATLAB Function/6(GPSLat), Distance/2(GPSLat)  "<latitude>"
  Bus Selector/7 -> MATLAB Function/7(GPSLong), Distance/3(GPSLong)  "<longitude>"
  Distance/1(Distance) -> Compare To Constant/1
  RGB image/1 -> Insert Text/1
  Insert Text/1 -> Output Heirarchy/1(Annotated Image)
  Data Type Conversion2/1 -> Output Heirarchy/5(Task Finished)
  Compare To Constant/1 -> Logical Operator/2
  MATLAB Function/3(gateGPS) -> Distance/1(DesiredGPS)
  Compare To Constant1/1 -> Logical Operator/1
  Logical Operator/1 -> Data Type Conversion2/1

== system RoboBoat_NEDcallv8/Main FSM/Obstacle Navigation1/Enter Gate/Gate 2 (White & White) ==
  Sensors : Inport
  RGB image : Inport  Port=2
  Enable : EnablePort  ShowOutputPort=on
  Bus Selector : BusSelector  OutputSignals=Serial In.Buoy Info.Probability,Serial In.Buoy Info.Color ID,Serial In.Buoy Info.Distance,Serial In.Buoy Info.Angle,Serial In.Compass.Heading,Serial In.GPS.latitude,Serial In.GPS.longitude
  Compare To Constant : simulink/Logic and Bit Operations/Compare To Constant  relop=<=  const=2  OutDataTypeStr=boolean
  Compare To Constant1 : simulink/Logic and Bit Operations/Compare To Constant  relop=>=  const=120  OutDataTypeStr=boolean
  Data Type Conversion2 : DataTypeConversion  OutDataTypeStr=double
  Discrete-Time Integrator : DiscreteIntegrator  SampleTime=.1  ICPrevOutput=DiscIntNeverNeededParam  ICPrevScaledInput=DiscIntNeverNeededParam
  Distance : MATLAB Function  TreatAsAtomicUnit=on
  Insert Text : visiontextngfix/Insert Text  inputType=Obsolete  theText='Enter Gate 2'  getTextLocFrom=Specify via dialog  textLoc=[1 1]  getTextColorFrom=Specify via dialog  textColor=[0 0 0]  getTextIntensityFrom=Specify via dialog  textIntensity=0  getTextOpacityFrom=Specify via dialog  textOpacity=1.0  dummyVar2=0  dummyVar3=0  dummyVar4=0  imagePorts=One multidimensional signal  isInputTransposed=off  fontFace=LucidaSansRegular  dummyVar1=0  blockFontSize=12  antiAliased=on
  Logical Operator : Logic  Operator=OR  AllPortsSameDT=off  OutDataTypeStr=boolean
  MATLAB Function : MATLAB Function  TreatAsAtomicUnit=on
  Output Heirarchy : Subsystem
  Outputs : Outport
  wires:
  Output Heirarchy/1(Outputs) -> Outputs/1
  Sensors/1 -> Output Heirarchy/2(Sensors), Bus Selector/1
  Bus Selector/1 -> MATLAB Function/1(Prob)  "<Probability>"
  Bus Selector/2 -> MATLAB Function/2(ColorID)  "<Color ID>"
  Bus Selector/3 -> MATLAB Function/3(Dist)  "<Distance>"
  Bus Selector/4 -> MATLAB Function/4(Ang)  "<Angle>"
  Bus Selector/5 -> MATLAB Function/5(CurrentHeading)  "<Heading>"
  Enable/1 -> Discrete-Time Integrator/1
  Discrete-Time Integrator/1 -> Compare To Constant1/1, MATLAB Function/8(Timer)
  MATLAB Function/1(RPM) -> Output Heirarchy/3(RPM)
  MATLAB Function/2(DesiredHeading) -> Output Heirarchy/4(Desired Heading)
  Bus Selector/6 -> MATLAB Function/6(GPSLat), Distance/2(GPSLat)  "<latitude>"
  Bus Selector/7 -> MATLAB Function/7(GPSLong), Distance/3(GPSLong)  "<longitude>"
  Distance/1(Distance) -> Compare To Constant/1
  RGB image/1 -> Insert Text/1
  Data Type Conversion2/1 -> Output Heirarchy/5(Task Finished)
  Compare To Constant/1 -> Logical Operator/2
  MATLAB Function/3(gateGPS) -> Distance/1(DesiredGPS)
  Compare To Constant1/1 -> Logical Operator/1
  Logical Operator/1 -> Data Type Conversion2/1
  Insert Text/1 -> Output Heirarchy/1(Annotated Image)

== system RoboBoat_NEDcallv8/Main FSM/Obstacle Navigation1/Enter Gate/Gate 3 (White & Green) ==
  Sensors : Inport
  RGB image : Inport  Port=2
  Enable : EnablePort  ShowOutputPort=on
  Bus Selector : BusSelector  OutputSignals=Serial In.Buoy Info.Probability,Serial In.Buoy Info.Color ID,Serial In.Buoy Info.Distance,Serial In.Buoy Info.Angle,Serial In.Compass.Heading,Serial In.GPS.latitude,Serial In.GPS.longitude
  Compare To Constant : simulink/Logic and Bit Operations/Compare To Constant  relop=<=  const=2  OutDataTypeStr=boolean
  Compare To Constant1 : simulink/Logic and Bit Operations/Compare To Constant  relop=>=  const=120  OutDataTypeStr=boolean
  Data Type Conversion2 : DataTypeConversion  OutDataTypeStr=double
  Discrete-Time Integrator : DiscreteIntegrator  SampleTime=.1  ICPrevOutput=DiscIntNeverNeededParam  ICPrevScaledInput=DiscIntNeverNeededParam
  Distance : MATLAB Function  TreatAsAtomicUnit=on
  Insert Text : visiontextngfix/Insert Text  inputType=Obsolete  theText='Enter Gate 3'  getTextLocFrom=Specify via dialog  textLoc=[1 1]  getTextColorFrom=Specify via dialog  textColor=[0 0 0]  getTextIntensityFrom=Specify via dialog  textIntensity=0  getTextOpacityFrom=Specify via dialog  textOpacity=1.0  dummyVar2=0  dummyVar3=0  dummyVar4=0  imagePorts=One multidimensional signal  isInputTransposed=off  fontFace=LucidaSansRegular  dummyVar1=0  blockFontSize=12  antiAliased=on
  Logical Operator : Logic  Operator=OR  AllPortsSameDT=off  OutDataTypeStr=boolean
  MATLAB Function : MATLAB Function  TreatAsAtomicUnit=on
  Output Heirarchy : Subsystem
  Outputs : Outport
  wires:
  Output Heirarchy/1(Outputs) -> Outputs/1
  Sensors/1 -> Output Heirarchy/2(Sensors), Bus Selector/1
  Bus Selector/1 -> MATLAB Function/1(Prob)  "<Probability>"
  Bus Selector/2 -> MATLAB Function/2(ColorID)  "<Color ID>"
  Bus Selector/3 -> MATLAB Function/3(Dist)  "<Distance>"
  Bus Selector/4 -> MATLAB Function/4(Ang)  "<Angle>"
  Bus Selector/5 -> MATLAB Function/5(CurrentHeading)  "<Heading>"
  Enable/1 -> Discrete-Time Integrator/1
  Discrete-Time Integrator/1 -> Compare To Constant1/1, MATLAB Function/8(Timer)
  MATLAB Function/1(RPM) -> Output Heirarchy/3(RPM)
  MATLAB Function/2(DesiredHeading) -> Output Heirarchy/4(Desired Heading)
  Bus Selector/6 -> MATLAB Function/6(GPSLat), Distance/2(GPSLat)  "<latitude>"
  Bus Selector/7 -> MATLAB Function/7(GPSLong), Distance/3(GPSLong)  "<longitude>"
  Distance/1(Distance) -> Compare To Constant/1
  RGB image/1 -> Insert Text/1
  Data Type Conversion2/1 -> Output Heirarchy/5(Task Finished)
  Compare To Constant/1 -> Logical Operator/2
  MATLAB Function/3(gateGPS) -> Distance/1(DesiredGPS)
  Compare To Constant1/1 -> Logical Operator/1
  Logical Operator/1 -> Data Type Conversion2/1
  Insert Text/1 -> Output Heirarchy/1(Annotated Image)

== system RoboBoat_NEDcallv8/Main FSM/Obstacle Navigation1/Enter Gate/Output Reassign ==
  Outputs in : Inport
  Bus Assignment : BusAssignment  AssignedSignals=Task Finished
  Bus Selector : BusSelector  OutputSignals=Task Finished
  Constant : Constant  Value=0
  Outputs : Outport
  Finished : Outport  Port=2
  wires:
  Outputs in/1 -> Bus Assignment/1, Bus Selector/1
  Bus Selector/1 -> Finished/1  "<Task Finished>"
  Bus Assignment/1 -> Outputs/1
  Constant/1 -> Bus Assignment/2

== system RoboBoat_NEDcallv8/Main FSM/Obstacle Navigation1/Exit Gate/Gate 1 (Red & White) ==
  Sensors : Inport
  RGB image : Inport  Port=2
  Enable : EnablePort  ShowOutputPort=on
  Bus Selector : BusSelector  OutputSignals=Serial In.Buoy Info.Probability,Serial In.Buoy Info.Color ID,Serial In.Buoy Info.Distance,Serial In.Buoy Info.Angle,Serial In.Compass.Heading,Serial In.GPS.latitude,Serial In.GPS.longitude
  Compare To Constant : simulink/Logic and Bit Operations/Compare To Constant  relop=<=  const=2  OutDataTypeStr=boolean
  Compare To Constant1 : simulink/Logic and Bit Operations/Compare To Constant  relop=>=  const=120  OutDataTypeStr=boolean
  Data Type Conversion2 : DataTypeConversion  OutDataTypeStr=double
  Discrete-Time Integrator : DiscreteIntegrator  SampleTime=.1  ICPrevOutput=DiscIntNeverNeededParam  ICPrevScaledInput=DiscIntNeverNeededParam
  Distance : MATLAB Function  TreatAsAtomicUnit=on
  Insert Text : visiontextngfix/Insert Text  inputType=Obsolete  theText='Exit Gate 1'  getTextLocFrom=Specify via dialog  textLoc=[1 1]  getTextColorFrom=Specify via dialog  textColor=[0 0 0]  getTextIntensityFrom=Specify via dialog  textIntensity=0  getTextOpacityFrom=Specify via dialog  textOpacity=1.0  dummyVar2=0  dummyVar3=0  dummyVar4=0  imagePorts=One multidimensional signal  isInputTransposed=off  fontFace=LucidaSansRegular  dummyVar1=0  blockFontSize=12  antiAliased=on
  Logical Operator : Logic  Operator=OR  AllPortsSameDT=off  OutDataTypeStr=boolean
  MATLAB Function : MATLAB Function  TreatAsAtomicUnit=on
  Output Heirarchy : Subsystem
  Outputs : Outport
  wires:
  Output Heirarchy/1(Outputs) -> Outputs/1
  Sensors/1 -> Output Heirarchy/2(Sensors), Bus Selector/1
  Bus Selector/1 -> MATLAB Function/1(Prob)  "<Probability>"
  Bus Selector/2 -> MATLAB Function/2(ColorID)  "<Color ID>"
  Bus Selector/3 -> MATLAB Function/3(Dist)  "<Distance>"
  Bus Selector/4 -> MATLAB Function/4(Ang)  "<Angle>"
  Bus Selector/5 -> MATLAB Function/5(CurrentHeading)  "<Heading>"
  Enable/1 -> Discrete-Time Integrator/1
  Discrete-Time Integrator/1 -> Compare To Constant1/1, MATLAB Function/8(Timer)
  MATLAB Function/1(RPM) -> Output Heirarchy/3(RPM)
  MATLAB Function/2(DesiredHeading) -> Output Heirarchy/4(Desired Heading)
  Bus Selector/6 -> MATLAB Function/6(GPSLat), Distance/2(GPSLat)  "<latitude>"
  Bus Selector/7 -> MATLAB Function/7(GPSLong), Distance/3(GPSLong)  "<longitude>"
  Distance/1(Distance) -> Compare To Constant/1
  RGB image/1 -> Insert Text/1
  Insert Text/1 -> Output Heirarchy/1(Annotated Image)
  Data Type Conversion2/1 -> Output Heirarchy/5(Task Finished)
  Compare To Constant/1 -> Logical Operator/2
  MATLAB Function/3(gateGPS) -> Distance/1(DesiredGPS)
  Compare To Constant1/1 -> Logical Operator/1
  Logical Operator/1 -> Data Type Conversion2/1

== system RoboBoat_NEDcallv8/Main FSM/Obstacle Navigation1/Exit Gate/Gate 2 (White & White) ==
  Sensors : Inport
  RGB image : Inport  Port=2
  Enable : EnablePort  ShowOutputPort=on
  Bus Selector : BusSelector  OutputSignals=Serial In.Buoy Info.Probability,Serial In.Buoy Info.Color ID,Serial In.Buoy Info.Distance,Serial In.Buoy Info.Angle,Serial In.Compass.Heading,Serial In.GPS.latitude,Serial In.GPS.longitude
  Compare To Constant : simulink/Logic and Bit Operations/Compare To Constant  relop=<=  const=2  OutDataTypeStr=boolean
  Compare To Constant1 : simulink/Logic and Bit Operations/Compare To Constant  relop=>=  const=120  OutDataTypeStr=boolean
  Data Type Conversion2 : DataTypeConversion  OutDataTypeStr=double
  Discrete-Time Integrator : DiscreteIntegrator  SampleTime=.1  ICPrevOutput=DiscIntNeverNeededParam  ICPrevScaledInput=DiscIntNeverNeededParam
  Distance : MATLAB Function  TreatAsAtomicUnit=on
  Insert Text : visiontextngfix/Insert Text  inputType=Obsolete  theText='Exit Gate 2'  getTextLocFrom=Specify via dialog  textLoc=[1 1]  getTextColorFrom=Specify via dialog  textColor=[0 0 0]  getTextIntensityFrom=Specify via dialog  textIntensity=0  getTextOpacityFrom=Specify via dialog  textOpacity=1.0  dummyVar2=0  dummyVar3=0  dummyVar4=0  imagePorts=One multidimensional signal  isInputTransposed=off  fontFace=LucidaSansRegular  dummyVar1=0  blockFontSize=12  antiAliased=on
  Logical Operator : Logic  Operator=OR  AllPortsSameDT=off  OutDataTypeStr=boolean
  MATLAB Function : MATLAB Function  TreatAsAtomicUnit=on
  Output Heirarchy : Subsystem
  Outputs : Outport
  wires:
  Output Heirarchy/1(Outputs) -> Outputs/1
  Sensors/1 -> Output Heirarchy/2(Sensors), Bus Selector/1
  Bus Selector/1 -> MATLAB Function/1(Prob)  "<Probability>"
  Bus Selector/2 -> MATLAB Function/2(ColorID)  "<Color ID>"
  Bus Selector/3 -> MATLAB Function/3(Dist)  "<Distance>"
  Bus Selector/4 -> MATLAB Function/4(Ang)  "<Angle>"
  Bus Selector/5 -> MATLAB Function/5(CurrentHeading)  "<Heading>"
  Enable/1 -> Discrete-Time Integrator/1
  Discrete-Time Integrator/1 -> Compare To Constant1/1, MATLAB Function/8(Timer)
  MATLAB Function/1(RPM) -> Output Heirarchy/3(RPM)
  MATLAB Function/2(DesiredHeading) -> Output Heirarchy/4(Desired Heading)
  Bus Selector/6 -> MATLAB Function/6(GPSLat), Distance/2(GPSLat)  "<latitude>"
  Bus Selector/7 -> MATLAB Function/7(GPSLong), Distance/3(GPSLong)  "<longitude>"
  Distance/1(Distance) -> Compare To Constant/1
  RGB image/1 -> Insert Text/1
  Data Type Conversion2/1 -> Output Heirarchy/5(Task Finished)
  Compare To Constant/1 -> Logical Operator/2
  MATLAB Function/3(gateGPS) -> Distance/1(DesiredGPS)
  Compare To Constant1/1 -> Logical Operator/1
  Logical Operator/1 -> Data Type Conversion2/1
  Insert Text/1 -> Output Heirarchy/1(Annotated Image)

== system RoboBoat_NEDcallv8/Main FSM/Obstacle Navigation1/Exit Gate/Gate 3 (White & Green) ==
  Sensors : Inport
  RGB image : Inport  Port=2
  Enable : EnablePort  ShowOutputPort=on
  Bus Selector : BusSelector  OutputSignals=Serial In.Buoy Info.Probability,Serial In.Buoy Info.Color ID,Serial In.Buoy Info.Distance,Serial In.Buoy Info.Angle,Serial In.Compass.Heading,Serial In.GPS.latitude,Serial In.GPS.longitude
  Compare To Constant : simulink/Logic and Bit Operations/Compare To Constant  relop=<=  const=2  OutDataTypeStr=boolean
  Compare To Constant1 : simulink/Logic and Bit Operations/Compare To Constant  relop=>=  const=120  OutDataTypeStr=boolean
  Data Type Conversion2 : DataTypeConversion  OutDataTypeStr=double
  Discrete-Time Integrator : DiscreteIntegrator  SampleTime=.1  ICPrevOutput=DiscIntNeverNeededParam  ICPrevScaledInput=DiscIntNeverNeededParam
  Distance : MATLAB Function  TreatAsAtomicUnit=on
  Insert Text : visiontextngfix/Insert Text  inputType=Obsolete  theText='Exit Gate 3'  getTextLocFrom=Specify via dialog  textLoc=[1 1]  getTextColorFrom=Specify via dialog  textColor=[0 0 0]  getTextIntensityFrom=Specify via dialog  textIntensity=0  getTextOpacityFrom=Specify via dialog  textOpacity=1.0  dummyVar2=0  dummyVar3=0  dummyVar4=0  imagePorts=One multidimensional signal  isInputTransposed=off  fontFace=LucidaSansRegular  dummyVar1=0  blockFontSize=12  antiAliased=on
  Logical Operator : Logic  Operator=OR  AllPortsSameDT=off  OutDataTypeStr=boolean
  MATLAB Function : MATLAB Function  TreatAsAtomicUnit=on
  Output Heirarchy : Subsystem
  Outputs : Outport
  wires:
  Output Heirarchy/1(Outputs) -> Outputs/1
  Sensors/1 -> Output Heirarchy/2(Sensors), Bus Selector/1
  Bus Selector/1 -> MATLAB Function/1(Prob)  "<Probability>"
  Bus Selector/2 -> MATLAB Function/2(ColorID)  "<Color ID>"
  Bus Selector/3 -> MATLAB Function/3(Dist)  "<Distance>"
  Bus Selector/4 -> MATLAB Function/4(Ang)  "<Angle>"
  Bus Selector/5 -> MATLAB Function/5(CurrentHeading)  "<Heading>"
  Enable/1 -> Discrete-Time Integrator/1
  Discrete-Time Integrator/1 -> Compare To Constant1/1, MATLAB Function/8(Timer)
  MATLAB Function/1(RPM) -> Output Heirarchy/3(RPM)
  MATLAB Function/2(DesiredHeading) -> Output Heirarchy/4(Desired Heading)
  Bus Selector/6 -> MATLAB Function/6(GPSLat), Distance/2(GPSLat)  "<latitude>"
  Bus Selector/7 -> MATLAB Function/7(GPSLong), Distance/3(GPSLong)  "<longitude>"
  Distance/1(Distance) -> Compare To Constant/1
  RGB image/1 -> Insert Text/1
  Data Type Conversion2/1 -> Output Heirarchy/5(Task Finished)
  Compare To Constant/1 -> Logical Operator/2
  MATLAB Function/3(gateGPS) -> Distance/1(DesiredGPS)
  Compare To Constant1/1 -> Logical Operator/1
  Logical Operator/1 -> Data Type Conversion2/1
  Insert Text/1 -> Output Heirarchy/1(Annotated Image)
